simulink model "lab"  (R2025b)
settings: Solver=VariableStepAuto  StartTime=0.0  StopTime=10.0  RelTol=1e-3
settings Model: Creator=mahesh  LastModifiedBy=mahesh

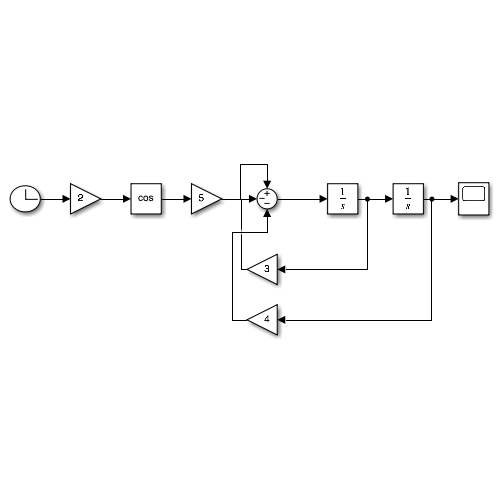
[thumbnail: Simulink's stored preview of the top-level diagram]
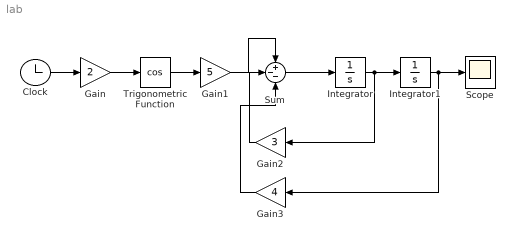
== system lab ==
  Clock : Clock
  Gain : Gain  Gain=2
  Gain1 : Gain  Gain=5
  Gain2 : Gain  Gain=3
  Gain3 : Gain  Gain=4
  Integrator : Integrator
  Integrator1 : Integrator
  Scope : Scope
      settings: ActiveDisplayYMinimum=-1.0428170792488909  ActiveDisplayYMaximum=1.0433409036682597
  Sum : Sum  Inputs=+--
  Trigonometric Function : Trigonometry  Operator=cos
  wires:
  Clock/1 -> Gain/1
  Gain/1 -> Trigonometric Function/1
  Trigonometric Function/1 -> Gain1/1
  Integrator/1 -> Gain2/1, Integrator1/1
  Sum/1 -> Integrator/1
  Gain1/1 -> Sum/1
  Integrator1/1 -> Gain3/1, Scope/1
  Gain2/1 -> Sum/2
  Gain3/1 -> Sum/3
